simulink model "Mdl_wAirbag"  (R2024b)
settings: Solver=FixedStepDiscrete  StartTime=0.0  StopTime=10.0  FixedStep=0.1  RelTol=1e-3  EnableMultiTasking=on
values from neighbouring files (symbols this model uses):
  AIRBAG_SYSTEM_STAT_OFF = mpt.Parameter    [Mdl_wAirbag_dd.m]
  AIRBAG_SYSTEM_STAT_ON = mpt.Parameter    [Mdl_wAirbag_dd.m]
  CAN_AIRBAG_SIGN_ONE_VALUE = mpt.Parameter    [Mdl_wAirbag_dd.m]
undefined symbols (not defined in the file or in its folder): CLUSTER_INACTIVE, eAirbagIn, eSIGNAL_MISSING, eSIGNAL_NEVER_RECEIVED, IgnOff, pJustRcvdStatus, RxCan_SignalClearJustRcvdStatus, RxCan_SignalGetJustRcvdStatus, RxCan_SignalInvalidProcessingControl, RxCan_SignalMissingProcessingControl, RxCan_SignalNRProcessingControl, SignalId, Status, tRxSignalId_type_instance, tRxSignalJustRcvdStatus_type_instance, tRxSignalStatus_type_instance, UI_WARNING_EVENT_NONE, UpdateWarningStatus, WarningCurEvent, WarningCurId, WarningCurStatus, WarningEvent_type_instance, WarningId_type_instance, WarningPayload, WarningStatus_type_instance, WRN_NORM_AIRBAG_03
settings Model: Creator=AELANGO6  LastModifiedBy=AELANGO6
settings DataIOCC: SaveOutput=off
settings OptimizationCC: DefaultParameterBehavior=Inlined  EnhancedBackFolding=on  PassReuseOutputArgsAs=Individual arguments  ZeroExternalMemoryAtStartup=off  ZeroInternalMemoryAtStartup=off  MaxStackSize=750  RemoveLocalVariableInitialization=off  OptimizeBlockOrder=speed  DifferentSizesBufferReuse=on  OptimizationCustomize=off  EfficientTunableParamExpr=on
settings DebuggingCC: ParameterTunabilityLossMsg=error
settings SFSimCC: MATLABDynamicMemAlloc=off
settings RTWCC: Description=AUTOSAR  SystemTargetFile=autosar.tlc  GenCodeOnly=on  TemplateMakefile=ert_default_tmf  PortableWordSizes=on  DataTypeReplacement=CDataTypesFixedWidth
settings CodeAppCC: ForceParamTrailComments=on  IgnoreCustomStorageClasses=off  OperatorAnnotations=on  SimulinkDataObjDesc=on  SFDataObjDesc=on  InsertBlockDesc=on
settings STFCustomTargetCC: TargetLangStandard=C99 (ISO)  MultiwordLength=256  ParMdlRefBuildCompliant=on  CompOptLevelCompliant=on  IncludeMdlTerminateFcn=off  CombineOutputUpdateFcns=on  SuppressErrorStatus=on  ERTCustomFileBanners=on  SupportNonFinite=off  SupportComplex=off  SupportContinuousTime=off  SupportNonInlinedSFcns=off  RemoveResetFunc=on  ParenthesesLevel=Maximum  CastingMode=Standards  MATLABClassNameForMDSCustomization=Simulink.SoftwareTarget.ERTCustomization  AutosarCompliant=on  UseToolchainInfoCompliant=on  LookupTableObjectStructAxisOrder=2,1,3,4,...  LUTObjectStructOrderEvenSpacing=Size,Table,Breakpoints  SystemTargetFile=autosar.tlc
settings ERTTargetCC: TargetLangStandard=C99 (ISO)  ConcurrentExecutionCompliant=off  IncludeMdlTerminateFcn=off  SuppressErrorStatus=on  SupportNonFinite=off  SupportComplex=off  ParenthesesLevel=Maximum  CastingMode=Standards  ModelStepFunctionPrototypeControlCompliant=off  CPPClassGenCompliant=off  AutosarCompliant=on  LookupTableObjectStructAxisOrder=2,1,3,4,...  LUTObjectStructOrderEvenSpacing=Size,Table,Breakpoints  ERTCustomFileTemplate=example_file_process.tlc  ERTFilePackagingFormat=CompactWithDataFile  BooleanTrueId=TRUE  BooleanFalseId=FALSE

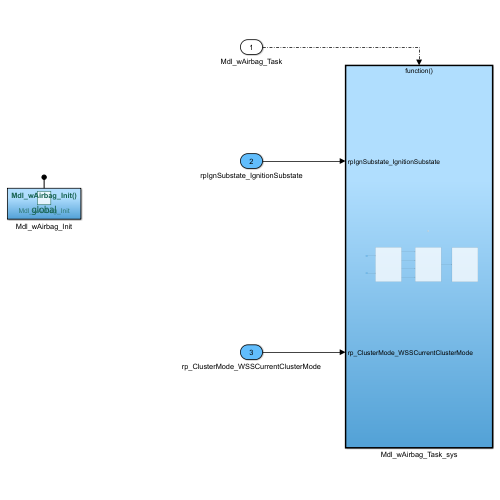
[thumbnail: Simulink's stored preview of the top-level diagram]
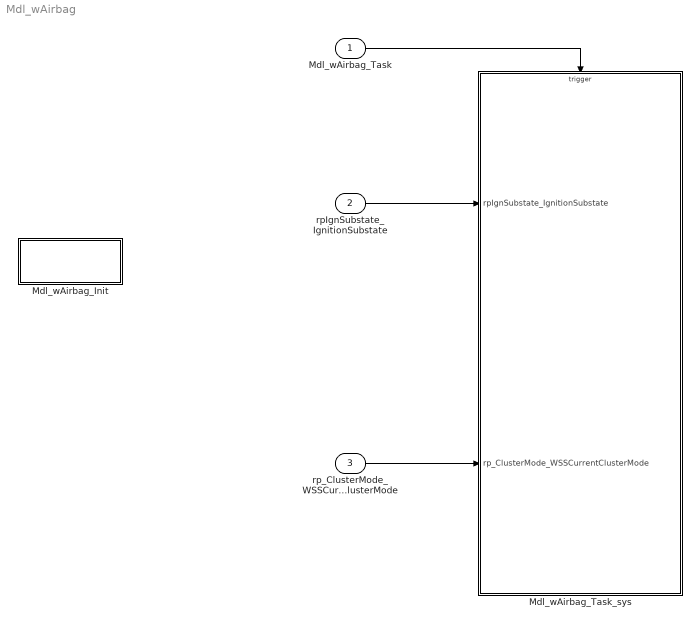
== system Mdl_wAirbag ==
  Mdl_wAirbag_Task : Inport  SampleTime=0.1  OutputFunctionCall=on
  rpIgnSubstate_IgnitionSubstate : Inport  Port=2  OutDataTypeStr=IgntionSubstateType  PortDimensions=1
  rp_ClusterMode_WSSCurrentClusterMode : Inport  Port=3  OutDataTypeStr=ClusterModes  PortDimensions=1
  Mdl_wAirbag_Init : Subsystem  TreatAsAtomicUnit=on
  Mdl_wAirbag_Task_sys : Subsystem  TreatAsAtomicUnit=on
  wires:
  rp_ClusterMode_WSSCurrentClusterMode/1 -> Mdl_wAirbag_Task_sys/2(rp_ClusterMode_WSSCurrentClusterMode)
  Mdl_wAirbag_Task/1 -> Mdl_wAirbag_Task_sys/Trigger
  rpIgnSubstate_IgnitionSubstate/1 -> Mdl_wAirbag_Task_sys/1(rpIgnSubstate_IgnitionSubstate)

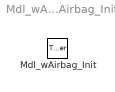
== system Mdl_wAirbag/Mdl_wAirbag_Init ==
  Mdl_wAirbag_Init : TriggerPort  TriggerType=function-call  IsSimulinkFunction=on  FunctionName=Mdl_wAirbag_Init  VariantControl=(inherit)

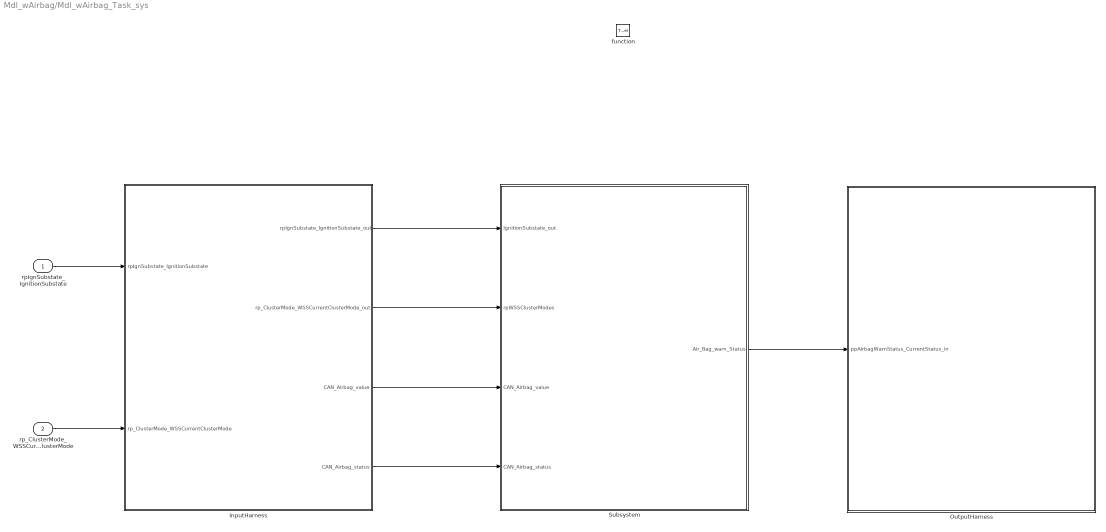
== system Mdl_wAirbag/Mdl_wAirbag_Task_sys ==
  rpIgnSubstate_IgnitionSubstate : Inport  OutDataTypeStr=IgntionSubstateType  PortDimensions=1
  rp_ClusterMode_WSSCurrentClusterMode : Inport  Port=2  OutDataTypeStr=ClusterModes  PortDimensions=1
  function : TriggerPort  TriggerType=function-call  VariantControl=(inherit)  SampleTimeType=periodic  SampleTime=-1
  InputHarness : Subsystem  Variant=on
  OutputHarness : Subsystem  Variant=on
  Subsystem : Subsystem
  wires:
  rpIgnSubstate_IgnitionSubstate/1 -> InputHarness/1(rpIgnSubstate_IgnitionSubstate)
  rp_ClusterMode_WSSCurrentClusterMode/1 -> InputHarness/2(rp_ClusterMode_WSSCurrentClusterMode)
  Subsystem/1(Air_Bag_warn_Status) -> OutputHarness/1(ppAirbagWarnStatus_CurrentStatus_in)
  InputHarness/1(rpIgnSubstate_IgnitionSubstate_out) -> Subsystem/1(IgnitionSubstate_out)
  InputHarness/2(rp_ClusterMode_WSSCurrentClusterMode_out) -> Subsystem/2(rpWSSClusterModes)
  InputHarness/3(CAN_Airbag_value) -> Subsystem/3(CAN_Airbag_value)
  InputHarness/4(CAN_Airbag_status) -> Subsystem/4(CAN_Airbag_status)

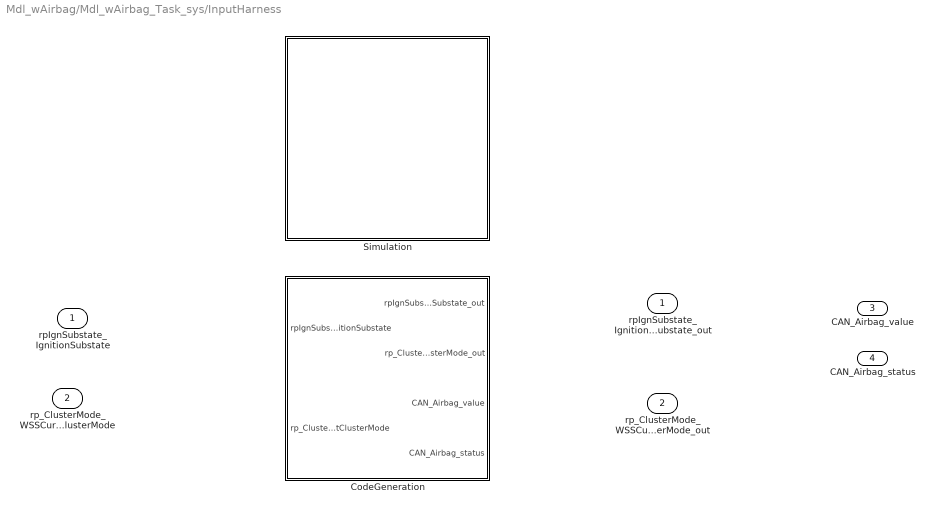
== system Mdl_wAirbag/Mdl_wAirbag_Task_sys/InputHarness ==
  rpIgnSubstate_IgnitionSubstate : Inport  OutDataTypeStr=IgntionSubstateType  PortDimensions=1
  rp_ClusterMode_WSSCurrentClusterMode : Inport  Port=2  OutDataTypeStr=ClusterModes  PortDimensions=1
  CodeGeneration : Subsystem  VariantControl=CODEGENERATION
  Simulation : Subsystem  VariantControl=SIMULATION
  rpIgnSubstate_IgnitionSubstate_out : Outport  OutDataTypeStr=IgntionSubstateType  PortDimensions=1
  rp_ClusterMode_WSSCurrentClusterMode_out : Outport  Port=2  OutDataTypeStr=ClusterModes  PortDimensions=1
  CAN_Airbag_value : Outport  Port=3  VectorParamsAs1DForOutWhenUnconnected=off
  CAN_Airbag_status : Outport  Port=4  VectorParamsAs1DForOutWhenUnconnected=off

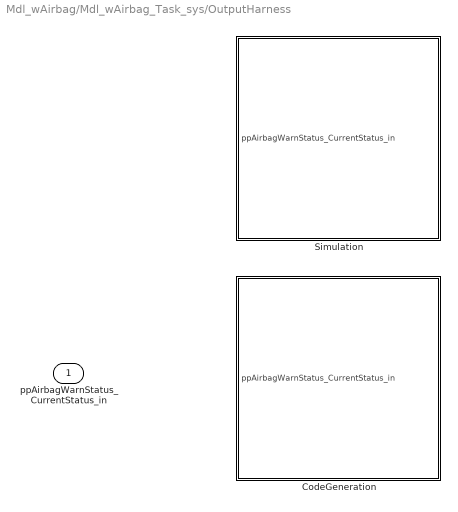
== system Mdl_wAirbag/Mdl_wAirbag_Task_sys/OutputHarness ==
  ppAirbagWarnStatus_CurrentStatus_in : Inport  PortDimensions=1
  CodeGeneration : Subsystem  VariantControl=CODEGENERATION
  Simulation : Subsystem  VariantControl=SIMULATION

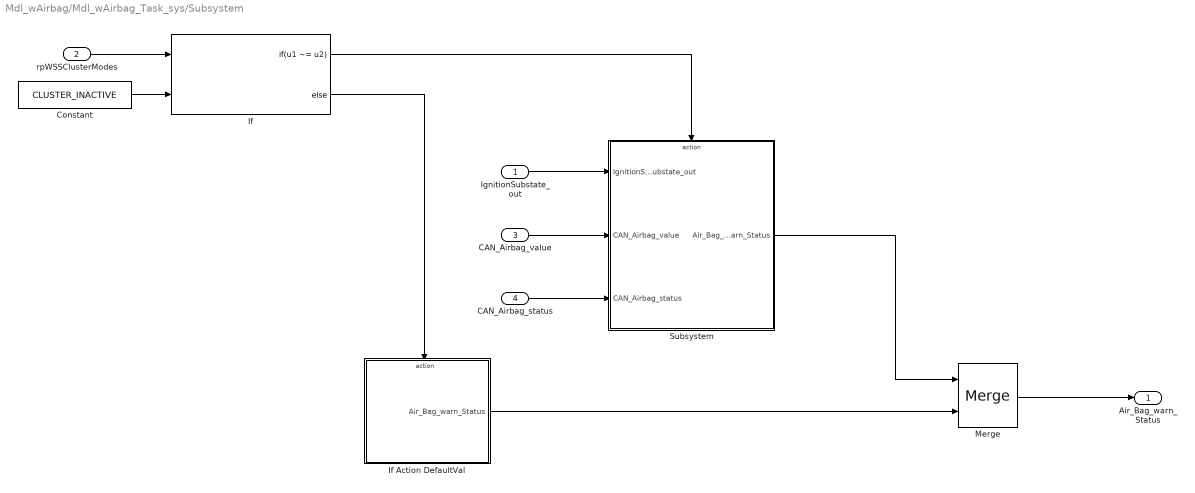
== system Mdl_wAirbag/Mdl_wAirbag_Task_sys/Subsystem ==
  IgnitionSubstate_out : Inport
  rpWSSClusterModes : Inport  Port=2
  CAN_Airbag_value : Inport  Port=3
  CAN_Airbag_status : Inport  Port=4
  Constant : Constant  Value=CLUSTER_INACTIVE
  If : If  NumInputs=2  IfExpression=u1 ~= u2
  If Action DefaultVal : Subsystem  TreatAsAtomicUnit=on
  Merge : Merge
  Subsystem : Subsystem
  Air_Bag_warn_Status : Outport  VectorParamsAs1DForOutWhenUnconnected=off
  wires:
  IgnitionSubstate_out/1 -> Subsystem/1(IgnitionSubstate_out)
  CAN_Airbag_value/1 -> Subsystem/2(CAN_Airbag_value)
  CAN_Airbag_status/1 -> Subsystem/3(CAN_Airbag_status)
  If/2 -> If Action DefaultVal/Action
  rpWSSClusterModes/1 -> If/1
  Constant/1 -> If/2
  If/1 -> Subsystem/Action
  Merge/1 -> Air_Bag_warn_Status/1
  If Action DefaultVal/1(Air_Bag_warn_Status) -> Merge/2
  Subsystem/1(Air_Bag_warn_Status) -> Merge/1

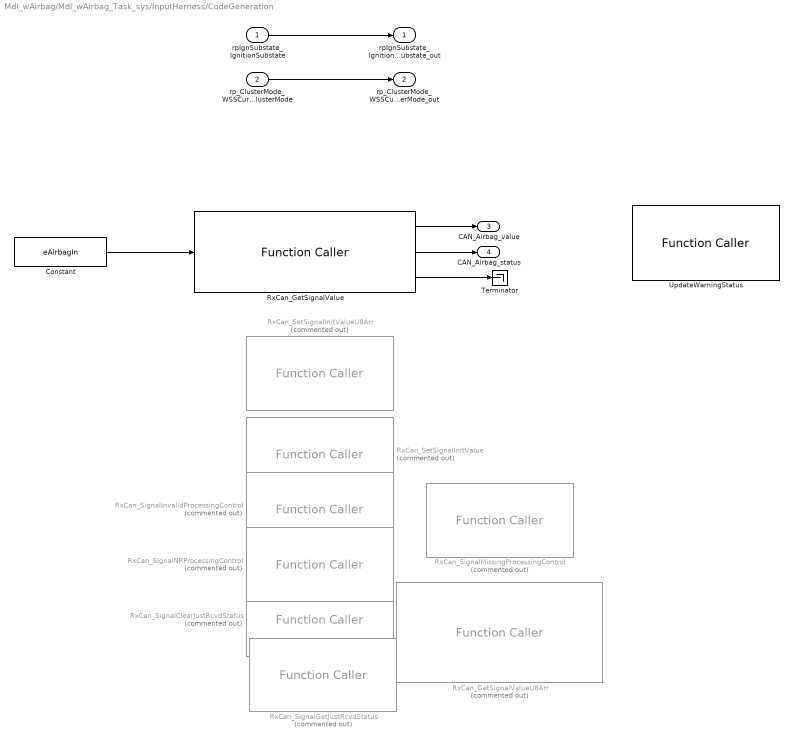
== system Mdl_wAirbag/Mdl_wAirbag_Task_sys/InputHarness/CodeGeneration ==
  rpIgnSubstate_IgnitionSubstate : Inport  OutDataTypeStr=IgntionSubstateType  PortDimensions=1
  rp_ClusterMode_WSSCurrentClusterMode : Inport  Port=2  OutDataTypeStr=ClusterModes  PortDimensions=1
  Constant : Constant  Value=eAirbagIn
  RxCan_GetSignalValue : FunctionCaller  FunctionPrototype=[pSignalValue,pSignalStatus,error_status] = RxCan_GetSignalValue(SignalId)  InputArgumentSpecifications=tRxSignalId_type_instance(1)  OutputArgumentSpecifications=uint8(1) ,tRxSignalStatus_type_instance(1) ,uint8(1)
  RxCan_GetSignalValueU8Arr : FunctionCaller  Commented=on  FunctionPrototype=[pSignalValue,pSignalStatus,pSignalLength,error_status] = RxCan_GetSignalValueU8Arr(SignalId)  InputArgumentSpecifications=tRxSignalId_type_instance(1)  OutputArgumentSpecifications=uint8(1) ,tRxSignalStatus_type_instance(1) ,uint32(1) ,uint8(1)
  RxCan_SetSignalInitValue : FunctionCaller  Commented=on  FunctionPrototype=[pSignalValue,error_status] = RxCan_SetSignalInitValue(SignalId)  InputArgumentSpecifications=tRxSignalId_type_instance(1)  OutputArgumentSpecifications=uint8(1) ,uint8(1)
  RxCan_SetSignalInitValueU8Arr : FunctionCaller  Commented=on  FunctionPrototype=[pSignaValue,pSignalLength,error_status] = RxCan_SetSignalInitValueU8Arr(SignalId)  InputArgumentSpecifications=tRxSignalId_type_instance(1)  OutputArgumentSpecifications=uint8(1) ,uint32(1) ,uint8(1)
  RxCan_SignalClearJustRcvdStatus : FunctionCaller  Commented=on  FunctionPrototype=RxCan_SignalClearJustRcvdStatus(SignalId)  InputArgumentSpecifications=tRxSignalId_type_instance(1)  OutputArgumentSpecifications=<Enter example>
  RxCan_SignalGetJustRcvdStatus : FunctionCaller  Commented=on  FunctionPrototype=RxCan_SignalGetJustRcvdStatus(SignalId,pJustRcvdStatus)  InputArgumentSpecifications=tRxSignalId_type_instance(1) ,tRxSignalJustRcvdStatus_type_instance(1)  OutputArgumentSpecifications=<Enter example>
  RxCan_SignalInvalidProcessingControl : FunctionCaller  Commented=on  FunctionPrototype=RxCan_SignalInvalidProcessingControl(SignalId,Status)  InputArgumentSpecifications=tRxSignalId_type_instance(1) ,boolean(1)  OutputArgumentSpecifications=<Enter example>
  RxCan_SignalMissingProcessingControl : FunctionCaller  Commented=on  FunctionPrototype=RxCan_SignalMissingProcessingControl(SignalId,Status)  InputArgumentSpecifications=tRxSignalId_type_instance(1) ,boolean(1)  OutputArgumentSpecifications=<Enter example>
  RxCan_SignalNRProcessingControl : FunctionCaller  Commented=on  FunctionPrototype=RxCan_SignalNRProcessingControl(SignalId,Status)  InputArgumentSpecifications=tRxSignalId_type_instance(1) ,boolean(1)  OutputArgumentSpecifications=<Enter example>
  Terminator : Terminator
  UpdateWarningStatus : FunctionCaller  FunctionPrototype=UpdateWarningStatus(WarningCurId,WarningCurStatus,WarningCurEvent,WarningPayload)  InputArgumentSpecifications=WarningId_type_instance(1) ,WarningStatus_type_instance(1) ,WarningEvent_type_instance(1) ,uint32(1)  OutputArgumentSpecifications=<Enter example>
  rpIgnSubstate_IgnitionSubstate_out : Outport  OutDataTypeStr=IgntionSubstateType  PortDimensions=1
  rp_ClusterMode_WSSCurrentClusterMode_out : Outport  Port=2  OutDataTypeStr=ClusterModes  PortDimensions=1
  CAN_Airbag_value : Outport  Port=3  VectorParamsAs1DForOutWhenUnconnected=off
  CAN_Airbag_status : Outport  Port=4  VectorParamsAs1DForOutWhenUnconnected=off
  wires:
  rpIgnSubstate_IgnitionSubstate/1 -> rpIgnSubstate_IgnitionSubstate_out/1
  rp_ClusterMode_WSSCurrentClusterMode/1 -> rp_ClusterMode_WSSCurrentClusterMode_out/1
  Constant/1 -> RxCan_GetSignalValue/1
  RxCan_GetSignalValue/3 -> Terminator/1
  RxCan_GetSignalValue/1 -> CAN_Airbag_value/1
  RxCan_GetSignalValue/2 -> CAN_Airbag_status/1

== system Mdl_wAirbag/Mdl_wAirbag_Task_sys/InputHarness/Simulation ==

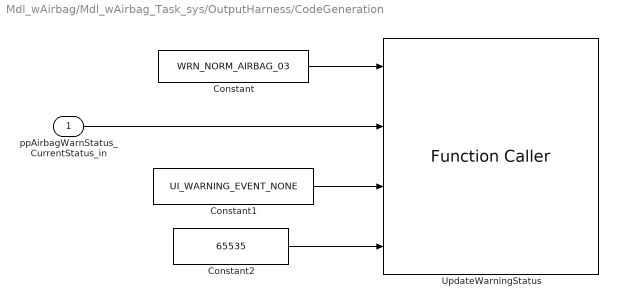
== system Mdl_wAirbag/Mdl_wAirbag_Task_sys/OutputHarness/CodeGeneration ==
  ppAirbagWarnStatus_CurrentStatus_in : Inport  PortDimensions=1
  Constant : Constant  Value=WRN_NORM_AIRBAG_03
  Constant1 : Constant  Value=UI_WARNING_EVENT_NONE
  Constant2 : Constant  Value=65535  OutDataTypeStr=uint32
  UpdateWarningStatus : FunctionCaller  FunctionPrototype=UpdateWarningStatus(WarningCurId,WarningCurStatus,WarningCurEvent,WarningPayload)  InputArgumentSpecifications=WarningId_type_instance(1) ,WarningStatus_type_instance(1) ,WarningEvent_type_instance(1) ,uint32(1)  OutputArgumentSpecifications=<Enter example>
  wires:
  ppAirbagWarnStatus_CurrentStatus_in/1 -> UpdateWarningStatus/2
  Constant/1 -> UpdateWarningStatus/1
  Constant1/1 -> UpdateWarningStatus/3
  Constant2/1 -> UpdateWarningStatus/4

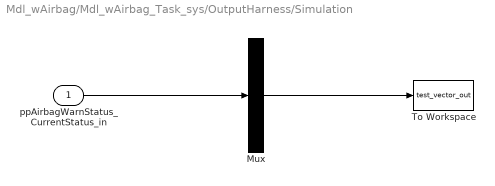
== system Mdl_wAirbag/Mdl_wAirbag_Task_sys/OutputHarness/Simulation ==
  ppAirbagWarnStatus_CurrentStatus_in : Inport  PortDimensions=1
  Mux : Mux  Inputs=1
  To Workspace : ToWorkspace  VariableName=test_vector_out  SaveFormat=Timeseries  SampleTime=-1
  wires:
  Mux/1 -> To Workspace/1
  ppAirbagWarnStatus_CurrentStatus_in/1 -> Mux/1

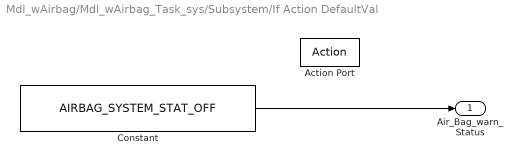
== system Mdl_wAirbag/Mdl_wAirbag_Task_sys/Subsystem/If Action DefaultVal ==
  Action Port : ActionPort  ActionPortLabel=else
  Constant : Constant  Value=AIRBAG_SYSTEM_STAT_OFF
  Air_Bag_warn_Status : Outport  VectorParamsAs1DForOutWhenUnconnected=off
  wires:
  Constant/1 -> Air_Bag_warn_Status/1

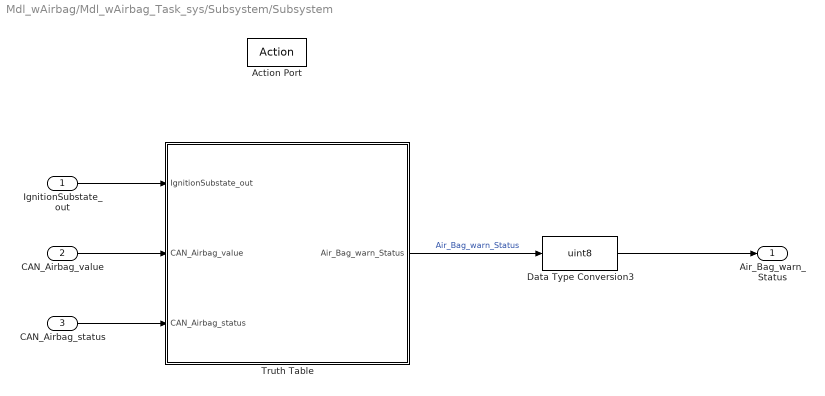
== system Mdl_wAirbag/Mdl_wAirbag_Task_sys/Subsystem/Subsystem ==
  IgnitionSubstate_out : Inport
  CAN_Airbag_value : Inport  Port=2
  CAN_Airbag_status : Inport  Port=3
  Action Port : ActionPort  ActionPortLabel=if(u1 ~= u2)
  Data Type Conversion3 : DataTypeConversion  OutDataTypeStr=uint8  SaturateOnIntegerOverflow=off  RndMeth=Floor
  Truth Table : Truth Table  TreatAsAtomicUnit=on
  Air_Bag_warn_Status : Outport  VectorParamsAs1DForOutWhenUnconnected=off
  wires:
  CAN_Airbag_status/1 -> Truth Table/3(CAN_Airbag_status)
  Truth Table/1(Air_Bag_warn_Status) -> Data Type Conversion3/1  "Air_Bag_warn_Status"
  Data Type Conversion3/1 -> Air_Bag_warn_Status/1
  IgnitionSubstate_out/1 -> Truth Table/1(IgnitionSubstate_out)
  CAN_Airbag_value/1 -> Truth Table/2(CAN_Airbag_value)

== matlab function Mdl_wAirbag/Mdl_wAirbag_Task_sys/Subsystem/Subsystem/Truth Table ==
  data: IgnitionSubstate_out input; Air_Bag_warn_Status output; CAN_Airbag_value input; CAN_Airbag_status input; CAN_AIRBAG_SIGN_ONE_VALUE parameter; eSIGNAL_MISSING parameter; eSIGNAL_NEVER_RECEIVED parameter double; IgnOff parameter; AIRBAG_SYSTEM_STAT_ON parameter; AIRBAG_SYSTEM_STAT_OFF parameter
function Air_Bag_warn_Status = fcn(IgnitionSubstate_out, CAN_Airbag_value, CAN_Airbag_status, CAN_AIRBAG_SIGN_ONE_VALUE, eSIGNAL_MISSING, eSIGNAL_NEVER_RECEIVED, IgnOff, AIRBAG_SYSTEM_STAT_ON, AIRBAG_SYSTEM_STAT_OFF)

aVarTruthTableCondition_1 = false;
aVarTruthTableCondition_2 = false;


% IGN ON Condition

aVarTruthTableCondition_1 = logical((IgnitionSubstate_out == IgnOff) ||  (CAN_Airbag_status == eSIGNAL_NEVER_RECEIVED));

% CAN Missing Condition

aVarTruthTableCondition_2 = logical((CAN_Airbag_status == eSIGNAL_MISSING) ||  (CAN_Airbag_value == CAN_AIRBAG_SIGN_ONE_VALUE));

if (aVarTruthTableCondition_1)
    aFcnTruthTableAction_1();
elseif (aVarTruthTableCondition_2)
    aFcnTruthTableAction_2();
else % Default
    aFcnTruthTableAction_1();
end

function aFcnTruthTableAction_1()

% AirBag Warning OFF Status

Air_Bag_warn_Status = AIRBAG_SYSTEM_STAT_OFF;

function aFcnTruthTableAction_2()

% AirBag Warning ON Status

Air_Bag_warn_Status = AIRBAG_SYSTEM_STAT_ON;
